simulink model "phi1_m2_vr001_k5_2"  (R2024b)
settings: Solver=FixedStepAuto  StartTime=0.0  StopTime=24.0  FixedStep=1.0  RelTol=1e-3
libraries: deeplib x1
settings Model: PacingRate=0.100000  Creator=ldy  LastModifiedBy=fedformi_new
settings DataIOCC: SaveFormat=Array  SignalLogging=off  DSMLogging=off  OutputOption=SpecifiedOutputTimes  OutputTimes=tspan

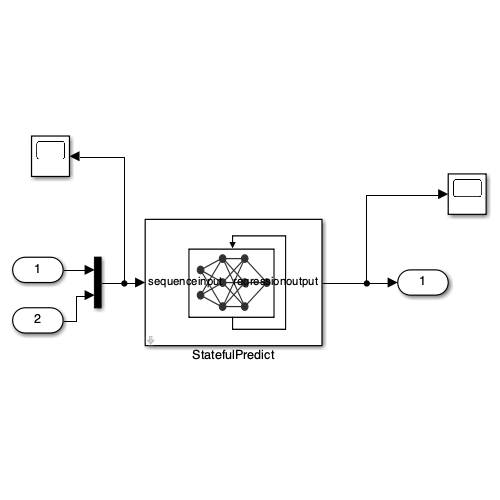
[thumbnail: Simulink's stored preview of the top-level diagram]
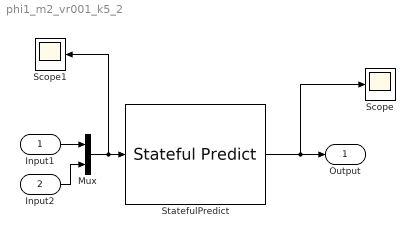
== system phi1_m2_vr001_k5_2 ==
  Input1 : Inport
  Input2 : Inport  Port=2
  Mux : Mux  Inputs=2
  Scope : Scope
  Scope1 : Scope
  StatefulPredict : deeplib/Stateful Predict  Network=Network from MAT-file  NetworkFunction=untitled  NetworkFilePath=SB1-Synthetic_Benchmark_1/phi1_m2_vr001_k5_2.mat  InputDataFormats={'',''}  SampleTime=1  ForceInterpretedSim=off  EnableDLNetwork=on  LastKnownNetworkFilePath=''  LastKnownNetworkTimeStamp=''
  Output : Outport
  wires:
  Input1/1 -> Mux/1
  Input2/1 -> Mux/2
  Mux/1 -> Scope1/1, StatefulPredict/1
  StatefulPredict/1 -> Scope/1, Output/1
